simulink model "Navigator"  (R2025b)
settings: Solver=FixedStepDiscrete  StartTime=0.0  StopTime=10  FixedStep=CMD_SAMPLE_TIME  RelTol=1e-3
undefined symbols (not defined in the file): CMD_SAMPLE_TIME, CMD_STOP_VELOCITY_TOLERANCE
libraries: simulink x1
settings Model: DataDictionary=CommandDict.sldd  Creator=89447  LastModifiedBy=89447
settings OptimizationCC: DefaultParameterBehavior=Inlined  EnhancedBackFolding=on  PassReuseOutputArgsAs=Individual arguments  ZeroExternalMemoryAtStartup=off  ZeroInternalMemoryAtStartup=off  MaxStackSize=64  OptimizeBlockOrder=speed  DifferentSizesBufferReuse=on  OptimizationCustomize=off  EfficientTunableParamExpr=on
settings HardwareCC: ProdBitPerLong=64.0  ProdHWDeviceType=Intel->x86-64 (Linux 64)  TargetBitPerLong=64.0  TargetBitPerPointer=64.0  TargetBitPerSizeT=64.0  TargetBitPerPtrDiffT=64.0  TargetLargestAtomicFloat=Float  TargetIntDivRoundTo=Zero  TargetEndianess=LittleEndian  TargetWordSize=64.0  TargetHWDeviceType=Intel->x86-64 (Linux 64)  ProdEqTarget=off
settings SFSimCC: MATLABDynamicMemAlloc=off
settings RTWCC: SystemTargetFile=ert.tlc  HardwareBoard=Robot Operating System 2 (ROS 2)  TLCOptions="-aInlineSetEventsForThisBaseRateFcn=TLC_FALSE -aSuppressMultiTaskScheduler=TLC_FALSE  -aRateBasedStepFcn=0"  TemplateMakefile=ert_default_tmf  Toolchain=Colcon Tools  TargetLang=C++  Description=Embedded Coder
settings CodeAppCC: ForceParamTrailComments=on  IgnoreCustomStorageClasses=off  OperatorAnnotations=on  SimulinkDataObjDesc=on  SFDataObjDesc=on  InsertBlockDesc=on
settings ERTTargetCC: ExtModeTransport=2.0  ExtModeStaticAlloc=on  ExtModeMexFile=ext_xcp  ExtModeIntrfLevel=Level2 - Open  ERTCustomFileTemplate=example_file_process.tlc  TargetLangStandard=C++11 (ISO)  SupportContinuousTime=on

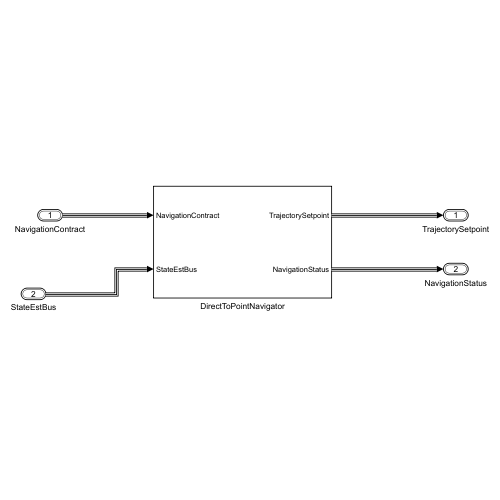
[thumbnail: Simulink's stored preview of the top-level diagram]
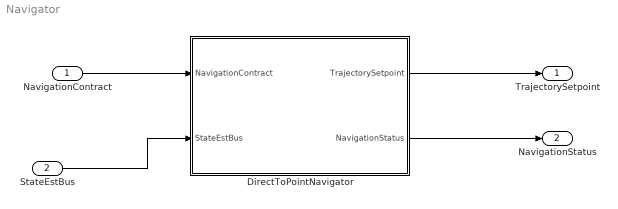
== system Navigator ==
  NavigationContract : Inport  OutDataTypeStr=Bus: NavigationContractBus
  StateEstBus : Inport  Port=2  OutDataTypeStr=Bus: StateEstBus
  DirectToPointNavigator : Subsystem
  TrajectorySetpoint : Outport  OutDataTypeStr=Bus: TrajectorySetpointBus
  NavigationStatus : Outport  Port=2  OutDataTypeStr=Bus: NavigationStatusBus
  wires:
  NavigationContract/1 -> DirectToPointNavigator/1(NavigationContract)
  StateEstBus/1 -> DirectToPointNavigator/2(StateEstBus)
  DirectToPointNavigator/1(TrajectorySetpoint) -> TrajectorySetpoint/1
  DirectToPointNavigator/2(NavigationStatus) -> NavigationStatus/1

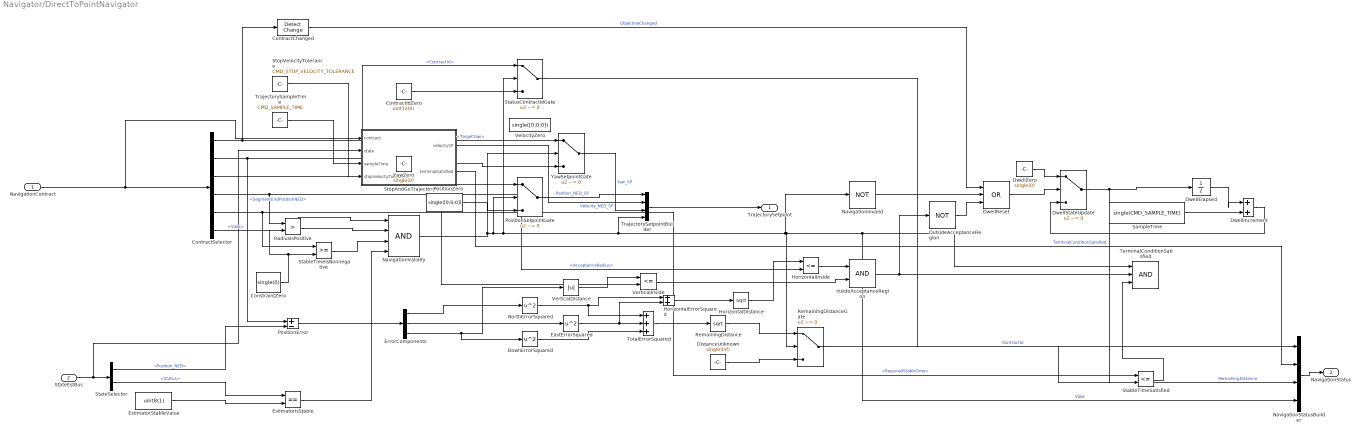
== system Navigator/DirectToPointNavigator ==
  NavigationContract : Inport  OutDataTypeStr=Bus: NavigationContractBus
  StateEstBus : Inport  Port=2  OutDataTypeStr=Bus: StateEstBus
  ConstraintZero : Constant  Value=single(0)
  ContractChanged : simulink/Logic and Bit Operations/Detect Change  vinit=uint32(0)  OutDataTypeStr=boolean
      settings: LibrarySourceBlock=|
      | hdlsllib/Logic and Bit
      | Operations/Detect
      | Change
  ContractIdZero : Constant  Value=uint32(0)
  ContractSelector : BusSelector  OutputSignals=ContractId,SegmentEndPositionNED,TargetYaw,AcceptanceRadius,RequiredStableTime,Valid
  DistanceUnknown : Constant  Value=single(inf)
  DownErrorSquared : Math  Operator=square
  DwellElapsed : UnitDelay  InitialCondition=single(0)  SampleTime=CMD_SAMPLE_TIME
  DwellIncrement : Sum  Inputs=|++
  DwellReset : Logic  Operator=OR  Inputs=3
  DwellStateUpdate : Switch  Criteria=u2 ~= 0
  DwellZero : Constant  Value=single(0)
  EastErrorSquared : Math  Operator=square
  ErrorComponents : Demux  Outputs=3
  EstimatorIsStable : RelationalOperator  Operator===
  EstimatorStableValue : Constant  Value=uint8(1)
  HorizontalDistance : Sqrt
  HorizontalErrorSquared : Sum  Inputs=|++
  HorizontalInside : RelationalOperator  Operator=<=
  InsideAcceptanceRegion : Logic
  NavigationInvalid : Logic  Operator=NOT
  NavigationStatusBuilder : BusCreator  Inputs=4
  NavigationValidity : Logic  Inputs=4
  NorthErrorSquared : Math  Operator=square
  OutsideAcceptanceRegion : Logic  Operator=NOT
  PositionError : Sum  Inputs=+-
  PositionSetpointGate : Switch  Criteria=u2 ~= 0
  PositionZero : Constant  Value=single([0;0;0])
  RadiusIsPositive : RelationalOperator  Operator=>
  RemainingDistance : Sqrt
  RemainingDistanceGate : Switch  Criteria=u2 ~= 0
  SampleTime : Constant  Value=single(CMD_SAMPLE_TIME)
  StableTimeIsNonnegative : RelationalOperator
  StableTimeSatisfied : RelationalOperator  Operator=<=
  StateSelector : BusSelector  OutputSignals=Position_NED,Status
  StatusContractIdGate : Switch  Criteria=u2 ~= 0
  StopAndGoTrajectory : MATLAB Function  TreatAsAtomicUnit=on
  StopVelocityTolerance : Constant  Value=CMD_STOP_VELOCITY_TOLERANCE  OutDataTypeStr=single
  TerminalConditionSatisfied : Logic  Inputs=3
  TotalErrorSquared : Sum  Inputs=+++
  TrajectorySampleTime : Constant  Value=CMD_SAMPLE_TIME  OutDataTypeStr=single
  TrajectorySetpointBuilder : BusCreator  Inputs=4
  VelocityZero : Constant  Value=single([0;0;0])
  VerticalDistance : Abs
  VerticalInside : RelationalOperator  Operator=<=
  YawSetpointGate : Switch  Criteria=u2 ~= 0
  YawZero : Constant  Value=single(0)
  TrajectorySetpoint : Outport  OutDataTypeStr=Bus: TrajectorySetpointBus
  NavigationStatus : Outport  Port=2  OutDataTypeStr=Bus: NavigationStatusBus
  wires:
  NavigationContract/1 -> StopAndGoTrajectory/1(contract), ContractSelector/1
  StateEstBus/1 -> StopAndGoTrajectory/2(state), StateSelector/1
  ContractSelector/2 -> PositionSetpointGate/1, PositionError/1  "<SegmentEndPositionNED>"
  StateSelector/1 -> PositionError/2  "<Position_NED>"
  PositionError/1 -> ErrorComponents/1
  ErrorComponents/1 -> NorthErrorSquared/1
  ErrorComponents/2 -> EastErrorSquared/1
  ErrorComponents/3 -> DownErrorSquared/1, VerticalDistance/1
  NorthErrorSquared/1 -> HorizontalErrorSquared/1, TotalErrorSquared/1
  EastErrorSquared/1 -> TotalErrorSquared/2, HorizontalErrorSquared/2
  DownErrorSquared/1 -> TotalErrorSquared/3
  StateSelector/2 -> EstimatorIsStable/1  "<Status>"
  EstimatorStableValue/1 -> EstimatorIsStable/2
  ContractSelector/4 -> HorizontalInside/2, VerticalInside/2, RadiusIsPositive/1  "<AcceptanceRadius>"
  ConstraintZero/1 -> RadiusIsPositive/2, StableTimeIsNonnegative/2
  ContractSelector/5 -> StableTimeIsNonnegative/1, StableTimeSatisfied/1  "<RequiredStableTime>"
  ContractSelector/6 -> NavigationValidity/1  "<Valid>"
  EstimatorIsStable/1 -> NavigationValidity/4
  RadiusIsPositive/1 -> NavigationValidity/2
  StableTimeIsNonnegative/1 -> NavigationValidity/3
  VerticalDistance/1 -> VerticalInside/1
  HorizontalInside/1 -> InsideAcceptanceRegion/1
  VerticalInside/1 -> InsideAcceptanceRegion/2
  ContractSelector/1 -> StatusContractIdGate/1, ContractChanged/1  "<ContractId>"
  DwellStateUpdate/1 -> DwellElapsed/1, StableTimeSatisfied/2
  DwellElapsed/1 -> DwellIncrement/1
  SampleTime/1 -> DwellIncrement/2
  NavigationValidity/1 -> YawSetpointGate/2, NavigationStatusBuilder/4, TerminalConditionSatisfied/1, RemainingDistanceGate/2, NavigationInvalid/1, TrajectorySetpointBuilder/4, StatusContractIdGate/2, PositionSetpointGate/2  "Valid"
  InsideAcceptanceRegion/1 -> TerminalConditionSatisfied/2, OutsideAcceptanceRegion/1
  NavigationInvalid/1 -> DwellReset/2
  OutsideAcceptanceRegion/1 -> DwellReset/3
  DwellZero/1 -> DwellStateUpdate/1
  DwellReset/1 -> DwellStateUpdate/2
  DwellIncrement/1 -> DwellStateUpdate/3
  StableTimeSatisfied/1 -> TerminalConditionSatisfied/3
  PositionZero/1 -> PositionSetpointGate/3
  ContractSelector/3 -> YawSetpointGate/1  "<TargetYaw>"
  YawZero/1 -> YawSetpointGate/3
  PositionSetpointGate/1 -> TrajectorySetpointBuilder/1  "Position_NED_SP"
  YawSetpointGate/1 -> TrajectorySetpointBuilder/3  "Yaw_SP"
  TrajectorySetpointBuilder/1 -> TrajectorySetpoint/1
  ContractIdZero/1 -> StatusContractIdGate/3
  DistanceUnknown/1 -> RemainingDistanceGate/3
  StatusContractIdGate/1 -> NavigationStatusBuilder/1  "ContractId"
  RemainingDistanceGate/1 -> NavigationStatusBuilder/3  "RemainingDistance"
  NavigationStatusBuilder/1 -> NavigationStatus/1
  HorizontalErrorSquared/1 -> HorizontalDistance/1
  HorizontalDistance/1 -> HorizontalInside/1
  TotalErrorSquared/1 -> RemainingDistance/1
  RemainingDistance/1 -> RemainingDistanceGate/1
  ContractChanged/1 -> DwellReset/1  "ObjectiveChanged"
  TrajectorySampleTime/1 -> StopAndGoTrajectory/3(sampleTime)
  StopVelocityTolerance/1 -> StopAndGoTrajectory/4(stopVelocityTolerance)
  StopAndGoTrajectory/1(velocitySP) -> TrajectorySetpointBuilder/2  "Velocity_NED_SP"
  StopAndGoTrajectory/2(terminalSatisfied) -> NavigationStatusBuilder/2  "TerminalConditionSatisfied"

== matlab function Navigator/DirectToPointNavigator/StopAndGoTrajectory ==
  data: contract input; velocitySP output; state input; sampleTime input; stopVelocityTolerance input; terminalSatisfied output
function [velocitySP, terminalSatisfied] = StopAndGoTrajectory(contract, state, sampleTime, stopVelocityTolerance)
%#codegen
persistent previousContractId previousVelocityCommand previousAccelerationCommand stableElapsed
velocitySP = zeros(3,1,'single');
terminalSatisfied = false;
if isempty(previousContractId)
    previousContractId = uint32(0);
    previousVelocityCommand = zeros(3,1,'single');
    previousAccelerationCommand = zeros(3,1,'single');
    stableElapsed = single(0);
end
valid = contract.Valid && state.Status == uint8(1) && sampleTime > single(0) && ...
    stopVelocityTolerance >= single(0) && contract.AcceptanceRadius > single(0) && ...
    contract.CruiseSpeed >= single(0) && contract.MaxAcceleration > single(0) && ...
    contract.MaxJerk > single(0);
if ~valid
    previousContractId = uint32(0);
    previousVelocityCommand(:) = single(0);
    previousAccelerationCommand(:) = single(0);
    stableElapsed = single(0);
    return
end
contractChanged = contract.ContractId ~= previousContractId;
if contractChanged
    previousContractId = contract.ContractId;
    previousVelocityCommand = single(state.Velocity_NED(:));
    previousAccelerationCommand(:) = single(0);
    stableElapsed = single(0);
end
positionError = single(contract.SegmentEndPositionNED(:)) - single(state.Position_NED(:));
remainingDistance = sqrt(sum(positionError .* positionError));
terminalVelocity = single(contract.TerminalVelocityNED(:));
desiredVelocity = terminalVelocity;
if remainingDistance > contract.AcceptanceRadius
    direction = positionError / max(remainingDistance, single(1.0e-6));
    brakingDistance = max(remainingDistance - contract.AcceptanceRadius, single(0));
    brakingSpeed = sqrt(single(2) * contract.MaxAcceleration * brakingDistance);
    targetSpeed = min(contract.CruiseSpeed, brakingSpeed);
    desiredVelocity = targetSpeed * direction;
end
desiredAcceleration = (desiredVelocity - previousVelocityCommand) / sampleTime;
desiredAcceleration = limitVector(desiredAcceleration, contract.MaxAcceleration);
desiredJerk = (desiredAcceleration - previousAccelerationCommand) / sampleTime;
limitedJerk = limitVector(desiredJerk, contract.MaxJerk);
accelerationCommand = previousAccelerationCommand + limitedJerk * sampleTime;
accelerationCommand = limitVector(accelerationCommand, contract.MaxAcceleration);
velocityCommand = previousVelocityCommand + accelerationCommand * sampleTime;
velocityCommand = limitVector(velocityCommand, contract.CruiseSpeed);
previousAccelerationCommand = accelerationCommand;
previousVelocityCommand = velocityCommand;
velocitySP = velocityCommand;
velocityError = single(state.Velocity_NED(:)) - terminalVelocity;
velocitySettled = sqrt(sum(velocityError .* velocityError)) <= stopVelocityTolerance;
positionSettled = remainingDistance <= contract.AcceptanceRadius;
if positionSettled && velocitySettled
    stableElapsed = stableElapsed + sampleTime;
else
    stableElapsed = single(0);
end
terminalSatisfied = positionSettled && velocitySettled && ...
    stableElapsed >= contract.RequiredStableTime;
end

function limited = limitVector(value, magnitudeLimit)
limited = single(value(:));
valueNorm = sqrt(sum(limited .* limited));
if valueNorm > magnitudeLimit && valueNorm > single(1.0e-6)
    limited = limited * (magnitudeLimit / valueNorm);
end
end
